simulink model "Unreal_Engine4"  (R2021a)
settings: Solver=ode14x  StartTime=0.0  StopTime=10.0  FixedStep=0.001  RelTol=1e-3
values from neighbouring files (symbols this model uses):
  env = read_environment_data    [main.m]
libraries: sim3dlib x28, simulink_extras x19, sim3dcameralib x1
settings Model: Creator=mojta  LastModifiedBy=mojta

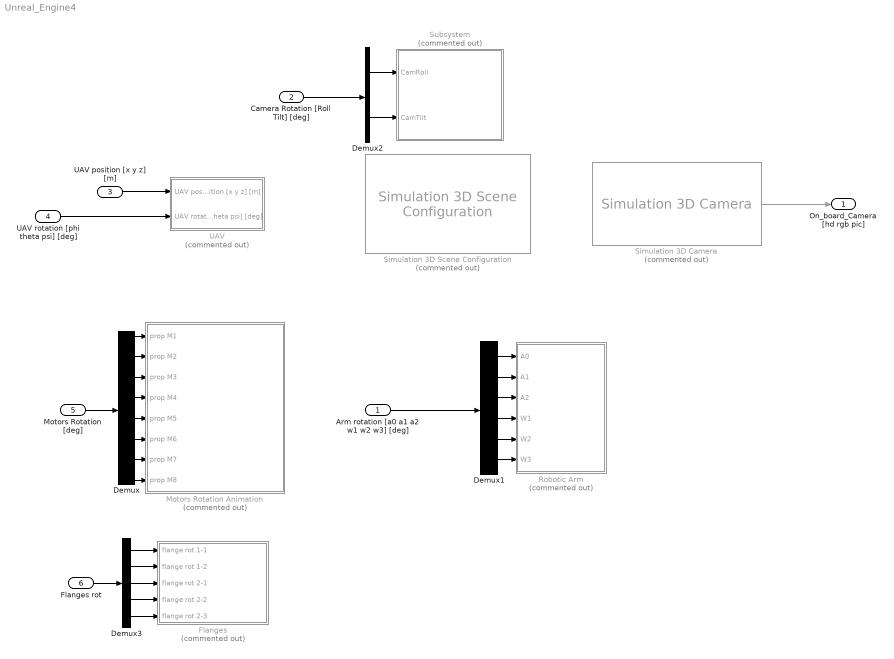
== system Unreal_Engine4 ==
  Arm rotation [a0 a1 a2 w1 w2 w3] [deg] : Inport  PortDimensions=6
  Camera Rotation [Roll Tilt] [deg] : Inport  Port=2  PortDimensions=2
  UAV position [x y z] [m] : Inport  Port=3  PortDimensions=3
  UAV rotation [phi theta psi] [deg] : Inport  Port=4  PortDimensions=3
  Motors Rotation [deg] : Inport  Port=5  PortDimensions=8
  Flanges rot : Inport  Port=6
  Demux : Demux  Outputs=8
  Demux1 : Demux  Outputs=6
  Demux2 : Demux  Outputs=2
  Demux3 : Demux  Outputs=5
  Flanges : Subsystem  Commented=on
  Motors Rotation Animation : Subsystem  Commented=on
  Robotic Arm : Subsystem  Commented=on
  Simulation 3D Camera : sim3dcameralib/Simulation 3D Camera  Priority=1  Commented=on  sensorTag=Sim3dSensor2  sensorId=2  sensorName=Sim3dSensor2  vehTagList={'Scene Origin'}  vehTag=Scene Origin  mountLoc=Origin  offsetFlag=on  tmountOffset=[0, 0, 0]  rmountOffset=[0 0 90]  FocalLength=[1109, 1109]  OpticalCenter=[640, 360]  ImageSize=[720, 1280]  RadialDistortion=[0, 0]  TangentialDistortion=[0, 0]  SensorSkew=0  DepthOutportEnabled=off  SemanticOutportEnabled=off  TransformOutportEnabled=off  SampleTime=1/160  mountPoint=[0 0 0]  mountOrientation=[0 0 -90]  aMode=3  ID=2
      settings: SourceProductBaseCode=DR,UV,VE
  Simulation 3D Scene Configuration : sim3dlib/Simulation 3D Scene Configuration  Priority=0  Commented=on  ProjectFormat=Unreal Editor  SceneDesc=Straight road  ProjectName=C:\Program Files\Polyspace\R2021a\toolbox\shared\sim3d_projects\automotive_project\UE4\WindowsNoEditor\VehicleSimulation.exe  ScenePath=/Game/Maps/HwStrght  UEProjPath=D:\MS_Control_Project\Sim_Env\Environment_1\Environment_1.uproject  vehTagList={'Scene Origin'}  vehTag=Scene Origin  OpVisEn=off  Ts=0.02  EnableWindow=on  EnableWeather=off  SunAltitude=40.0  SunAzimuth=90  clouds=10  wind=1  fog=0  rain=0  sensorTag=MainCamera1  sensorId=1  sensorName=MainCamera1  mountLoc=Origin  offsetFlag=off  tmountOffset=[0, 0, 0]  rmountOffset=[0, 0, 0]  HorizontalResolution=1280  VerticalResolution=720  HorizontalFOV=60  mountPoint=[0 0 0]  mountOrientation=[0 0 0]  aMode=2  ID=1
      settings: SourceProductBaseCode=DR,UV,VE
  Subsystem : Subsystem  Commented=on
  UAV : Subsystem  Commented=on
  On_board_Camera [hd rgb pic] : Outport  PortDimensions=[1280 720 3]
  wires:
  Simulation 3D Camera/1 -> On_board_Camera [hd rgb pic]/1
  Demux1/1 -> Robotic Arm/1(A0)
  Demux2/2 -> Subsystem/2(CamTilt)
  Demux1/3 -> Robotic Arm/3(A2)
  Demux1/5 -> Robotic Arm/5(W2)
  Demux2/1 -> Subsystem/1(CamRoll)
  Demux/5 -> Motors Rotation Animation/5(prop M5)
  Demux/7 -> Motors Rotation Animation/7(prop M7)
  Demux/3 -> Motors Rotation Animation/3(prop M3)
  Demux/1 -> Motors Rotation Animation/1(prop M1)
  Demux/2 -> Motors Rotation Animation/2(prop M2)
  Demux/4 -> Motors Rotation Animation/4(prop M4)
  Demux/6 -> Motors Rotation Animation/6(prop M6)
  Demux/8 -> Motors Rotation Animation/8(prop M8)
  Motors Rotation [deg]/1 -> Demux/1
  UAV position [x y z] [m]/1 -> UAV/1(UAV position [x y z] [m])
  UAV rotation [phi theta psi] [deg]/1 -> UAV/2(UAV rotation [phi theta psi] [deg])
  Demux1/2 -> Robotic Arm/2(A1)
  Demux1/4 -> Robotic Arm/4(W1)
  Demux1/6 -> Robotic Arm/6(W3)
  Arm rotation [a0 a1 a2 w1 w2 w3] [deg]/1 -> Demux1/1
  Camera Rotation [Roll Tilt] [deg]/1 -> Demux2/1
  Demux3/1 -> Flanges/1(flange rot 1-1)
  Demux3/2 -> Flanges/2(flange rot 1-2)
  Demux3/3 -> Flanges/3(flange rot 2-1)
  Demux3/4 -> Flanges/4(flange rot 2-2)
  Demux3/5 -> Flanges/5(flange rot 2-3)
  Flanges rot/1 -> Demux3/1

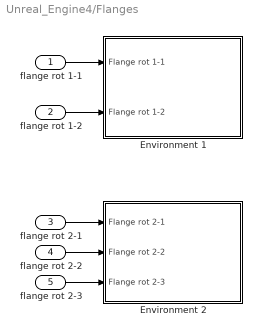
== system Unreal_Engine4/Flanges ==
  flange rot 1-1 : Inport  PortDimensions=8
  flange rot 1-2 : Inport  Port=2  PortDimensions=8
  flange rot 2-1 : Inport  Port=3  PortDimensions=6
  flange rot 2-2 : Inport  Port=4  PortDimensions=6
  flange rot 2-3 : Inport  Port=5  PortDimensions=6
  Environment 1 : Subsystem  TreatAsAtomicUnit=on
  Environment 2 : Subsystem  TreatAsAtomicUnit=on
  wires:
  flange rot 2-2/1 -> Environment 2/2(Flange rot 2-2)
  flange rot 2-3/1 -> Environment 2/3(Flange rot 2-3)
  flange rot 1-1/1 -> Environment 1/1(Flange rot 1-1)
  flange rot 1-2/1 -> Environment 1/2(Flange rot 1-2)
  flange rot 2-1/1 -> Environment 2/1(Flange rot 2-1)

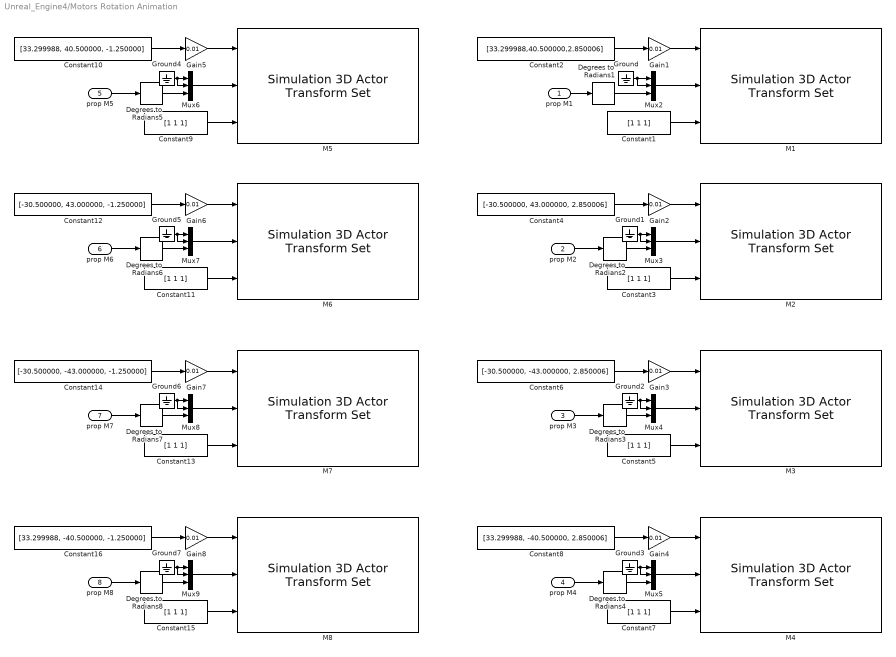
== system Unreal_Engine4/Motors Rotation Animation ==
  prop M1 : Inport
  prop M2 : Inport  Port=2
  prop M3 : Inport  Port=3
  prop M4 : Inport  Port=4
  prop M5 : Inport  Port=5
  prop M6 : Inport  Port=6
  prop M7 : Inport  Port=7
  prop M8 : Inport  Port=8
  Constant{1,3,5,7,9,11,13,15} (8 alike) : Constant  Value=[1 1 1]
  Constant10 : Constant  Value=[33.299988, 40.500000, -1.250000]
  Constant12 : Constant  Value=[-30.500000, 43.000000, -1.250000]
  Constant14 : Constant  Value=[-30.500000, -43.000000, -1.250000]
  Constant16 : Constant  Value=[33.299988, -40.500000, -1.250000]
  Constant2 : Constant  Value=[33.299988,40.500000,2.850006]
  Constant4 : Constant  Value=[-30.500000, 43.000000, 2.850006]
  Constant6 : Constant  Value=[-30.500000, -43.000000, 2.850006]
  Constant8 : Constant  Value=[33.299988, -40.500000, 2.850006]
  Degrees to Radians{1..8} (8 alike) : simulink_extras/Transformations/Degrees to Radians
  Gain{1..8} (8 alike) : Gain  Gain=0.01
  Ground{,1..7} (8 alike) : Ground
  M1 : sim3dlib/Simulation 3D Actor Transform Set  Priority=-1  ActorTag=M1  NumberOfParts=1  CustNumOfParts=3  Translation=[0 0 0]  Rotation=[0 0 0]  Scale=[1 1 1]  Ts=-1  aMode=2
      settings: SourceProductBaseCode=DR,UV,VE
  M2 : sim3dlib/Simulation 3D Actor Transform Set  Priority=-1  ActorTag=M2  NumberOfParts=1  CustNumOfParts=3  Translation=[0 0 0]  Rotation=[0 0 0]  Scale=[1 1 1]  Ts=-1  aMode=2
      settings: SourceProductBaseCode=DR,UV,VE
  M3 : sim3dlib/Simulation 3D Actor Transform Set  Priority=-1  ActorTag=M3  NumberOfParts=1  CustNumOfParts=3  Translation=[0 0 0]  Rotation=[0 0 0]  Scale=[1 1 1]  Ts=-1  aMode=2
      settings: SourceProductBaseCode=DR,UV,VE
  M4 : sim3dlib/Simulation 3D Actor Transform Set  Priority=-1  ActorTag=M4  NumberOfParts=1  CustNumOfParts=3  Translation=[0 0 0]  Rotation=[0 0 0]  Scale=[1 1 1]  Ts=-1  aMode=2
      settings: SourceProductBaseCode=DR,UV,VE
  M5 : sim3dlib/Simulation 3D Actor Transform Set  Priority=-1  ActorTag=M5  NumberOfParts=1  CustNumOfParts=3  Translation=[0 0 0]  Rotation=[0 0 0]  Scale=[1 1 1]  Ts=-1  aMode=2
      settings: SourceProductBaseCode=DR,UV,VE
  M6 : sim3dlib/Simulation 3D Actor Transform Set  Priority=-1  ActorTag=M6  NumberOfParts=1  CustNumOfParts=3  Translation=[0 0 0]  Rotation=[0 0 0]  Scale=[1 1 1]  Ts=-1  aMode=2
      settings: SourceProductBaseCode=DR,UV,VE
  M7 : sim3dlib/Simulation 3D Actor Transform Set  Priority=-1  ActorTag=M7  NumberOfParts=1  CustNumOfParts=3  Translation=[0 0 0]  Rotation=[0 0 0]  Scale=[1 1 1]  Ts=-1  aMode=2
      settings: SourceProductBaseCode=DR,UV,VE
  M8 : sim3dlib/Simulation 3D Actor Transform Set  Priority=-1  ActorTag=M8  NumberOfParts=1  CustNumOfParts=3  Translation=[0 0 0]  Rotation=[0 0 0]  Scale=[1 1 1]  Ts=-1  aMode=2
      settings: SourceProductBaseCode=DR,UV,VE
  Mux{2..9} (8 alike) : Mux  Inputs=3
  wires:
  Ground7/1 -> Mux9/1, Mux9/2
  Mux9/1 -> M8/2
  Constant7/1 -> M4/3
  Constant1/1 -> M1/3
  Gain8/1 -> M8/1
  Constant15/1 -> M8/3
  Constant16/1 -> Gain8/1
  Ground5/1 -> Mux7/2, Mux7/1
  prop M5/1 -> Degrees to Radians5/1
  Constant12/1 -> Gain6/1
  Constant6/1 -> Gain3/1
  prop M7/1 -> Degrees to Radians7/1
  Degrees to Radians1/1 -> Mux2/3
  Mux5/1 -> M4/2
  prop M2/1 -> Degrees to Radians2/1
  prop M4/1 -> Degrees to Radians4/1
  Gain7/1 -> M7/1
  Constant11/1 -> M6/3
  Degrees to Radians7/1 -> Mux8/3
  Mux8/1 -> M7/2
  Degrees to Radians6/1 -> Mux7/3
  Constant5/1 -> M3/3
  Mux4/1 -> M3/2
  Constant13/1 -> M7/3
  Gain1/1 -> M1/1
  Mux7/1 -> M6/2
  prop M3/1 -> Degrees to Radians3/1
  Constant14/1 -> Gain7/1
  prop M6/1 -> Degrees to Radians6/1
  Mux6/1 -> M5/2
  Gain6/1 -> M6/1
  Gain5/1 -> M5/1
  Degrees to Radians5/1 -> Mux6/3
  Degrees to Radians2/1 -> Mux3/3
  Gain3/1 -> M3/1
  Constant10/1 -> Gain5/1
  Constant8/1 -> Gain4/1
  Constant9/1 -> M5/3
  Constant4/1 -> Gain2/1
  Ground1/1 -> Mux3/2, Mux3/1
  Ground6/1 -> Mux8/1, Mux8/2
  Constant2/1 -> Gain1/1
  Ground4/1 -> Mux6/2, Mux6/1
  Ground3/1 -> Mux5/2, Mux5/1
  Ground/1 -> Mux2/2, Mux2/1
  Constant3/1 -> M2/3
  Ground2/1 -> Mux4/2, Mux4/1
  prop M8/1 -> Degrees to Radians8/1
  Mux3/1 -> M2/2
  Gain2/1 -> M2/1
  prop M1/1 -> Degrees to Radians1/1
  Mux2/1 -> M1/2
  Gain4/1 -> M4/1
  Degrees to Radians8/1 -> Mux9/3
  Degrees to Radians3/1 -> Mux4/3
  Degrees to Radians4/1 -> Mux5/3

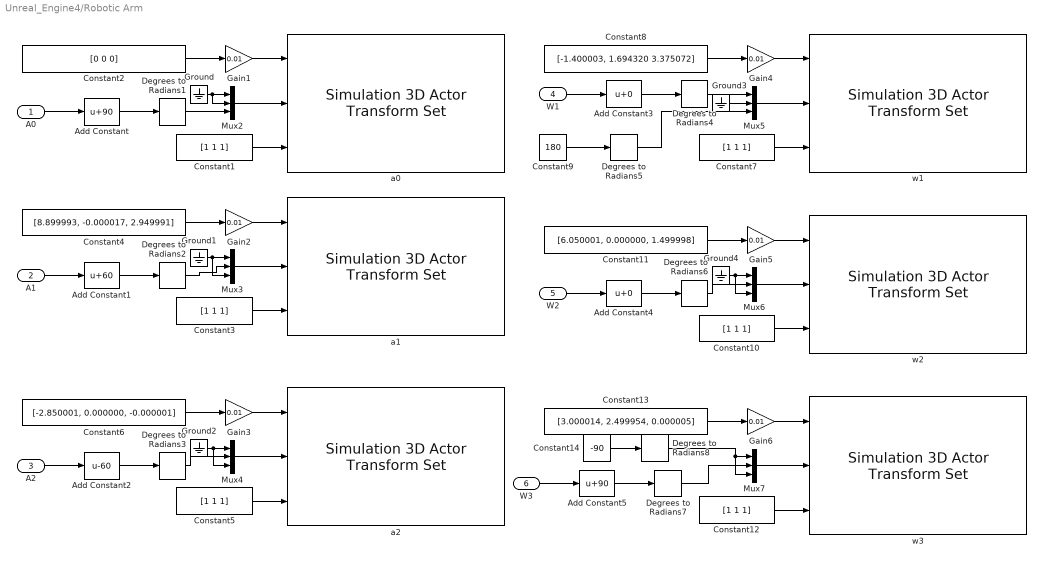
== system Unreal_Engine4/Robotic Arm ==
  A0 : Inport
  A1 : Inport  Port=2
  A2 : Inport  Port=3
  W1 : Inport  Port=4
  W2 : Inport  Port=5
  W3 : Inport  Port=6
  Add Constant : Bias  Bias=90
  Add Constant1 : Bias  Bias=60
  Add Constant2 : Bias  Bias=-60
  Add Constant3 : Bias
  Add Constant4 : Bias
  Add Constant5 : Bias  Bias=90
  Constant{1,3,5,7,10,12} (6 alike) : Constant  Value=[1 1 1]
  Constant11 : Constant  Value=[6.050001, 0.000000, 1.499998]
  Constant13 : Constant  Value=[3.000014, 2.499954, 0.000005]
  Constant14 : Constant  Value=-90
  Constant2 : Constant  Value=[0 0 0]
  Constant4 : Constant  Value=[8.899993, -0.000017, 2.949991]
  Constant6 : Constant  Value=[-2.850001, 0.000000, -0.000001]
  Constant8 : Constant  Value=[-1.400003, 1.694320 3.375072]
  Constant9 : Constant  Value=180
  Degrees to Radians{1..8} (8 alike) : simulink_extras/Transformations/Degrees to Radians
  Gain{1..6} (6 alike) : Gain  Gain=0.01
  Ground{,1..4} (5 alike) : Ground
  Mux{2..7} (6 alike) : Mux  Inputs=3
  a0 : sim3dlib/Simulation 3D Actor Transform Set  Priority=-1  ActorTag=A0  NumberOfParts=1  CustNumOfParts=3  Translation=[0 0 0]  Rotation=[0 0 0]  Scale=[1 1 1]  Ts=-1  aMode=2
      settings: SourceProductBaseCode=DR,UV,VE
  a1 : sim3dlib/Simulation 3D Actor Transform Set  Priority=-1  ActorTag=A1  NumberOfParts=1  CustNumOfParts=3  Translation=[0 0 0]  Rotation=[0 0 0]  Scale=[1 1 1]  Ts=-1  aMode=2
      settings: SourceProductBaseCode=DR,UV,VE
  a2 : sim3dlib/Simulation 3D Actor Transform Set  Priority=-1  ActorTag=A2  NumberOfParts=1  CustNumOfParts=3  Translation=[0 0 0]  Rotation=[0 0 0]  Scale=[1 1 1]  Ts=-1  aMode=2
      settings: SourceProductBaseCode=DR,UV,VE
  w1 : sim3dlib/Simulation 3D Actor Transform Set  Priority=-1  ActorTag=W1  NumberOfParts=1  CustNumOfParts=3  Translation=[0 0 0]  Rotation=[0 0 0]  Scale=[1 1 1]  Ts=-1  aMode=2
      settings: SourceProductBaseCode=DR,UV,VE
  w2 : sim3dlib/Simulation 3D Actor Transform Set  Priority=-1  ActorTag=W2  NumberOfParts=1  CustNumOfParts=3  Translation=[0 0 0]  Rotation=[0 0 0]  Scale=[1 1 1]  Ts=-1  aMode=2
      settings: SourceProductBaseCode=DR,UV,VE
  w3 : sim3dlib/Simulation 3D Actor Transform Set  Priority=-1  ActorTag=W3  NumberOfParts=1  CustNumOfParts=3  Translation=[0 0 0]  Rotation=[0 0 0]  Scale=[1 1 1]  Ts=-1  aMode=2
      settings: SourceProductBaseCode=DR,UV,VE
  wires:
  Constant7/1 -> w1/3
  Degrees to Radians2/1 -> Mux3/2
  W1/1 -> Add Constant3/1
  Mux3/1 -> a1/2
  Ground3/1 -> Mux5/2
  Constant14/1 -> Degrees to Radians8/1
  Gain4/1 -> w1/1
  Constant9/1 -> Degrees to Radians5/1
  Ground/1 -> Mux2/2, Mux2/1
  Degrees to Radians4/1 -> Mux5/1
  Constant8/1 -> Gain4/1
  Add Constant3/1 -> Degrees to Radians4/1
  Mux5/1 -> w1/2
  Mux7/1 -> w3/2
  Constant2/1 -> Gain1/1
  Degrees to Radians8/1 -> Mux7/1, Mux7/3
  Degrees to Radians1/1 -> Mux2/3
  Add Constant/1 -> Degrees to Radians1/1
  Constant1/1 -> a0/3
  Constant5/1 -> a2/3
  Mux6/1 -> w2/2
  Constant6/1 -> Gain3/1
  Mux2/1 -> a0/2
  Gain1/1 -> a0/1
  W2/1 -> Add Constant4/1
  Ground4/1 -> Mux6/3, Mux6/1
  Constant4/1 -> Gain2/1
  Constant11/1 -> Gain5/1
  Constant3/1 -> a1/3
  Add Constant4/1 -> Degrees to Radians6/1
  Mux4/1 -> a2/2
  Constant12/1 -> w3/3
  Degrees to Radians7/1 -> Mux7/2
  Constant13/1 -> Gain6/1
  W3/1 -> Add Constant5/1
  Add Constant2/1 -> Degrees to Radians3/1
  Gain6/1 -> w3/1
  Add Constant5/1 -> Degrees to Radians7/1
  A0/1 -> Add Constant/1
  Degrees to Radians3/1 -> Mux4/2
  A2/1 -> Add Constant2/1
  Gain5/1 -> w2/1
  Add Constant1/1 -> Degrees to Radians2/1
  Constant10/1 -> w2/3
  Gain2/1 -> a1/1
  Ground1/1 -> Mux3/3, Mux3/1
  Degrees to Radians5/1 -> Mux5/3
  Ground2/1 -> Mux4/3, Mux4/1
  Gain3/1 -> a2/1
  A1/1 -> Add Constant1/1
  Degrees to Radians6/1 -> Mux6/2

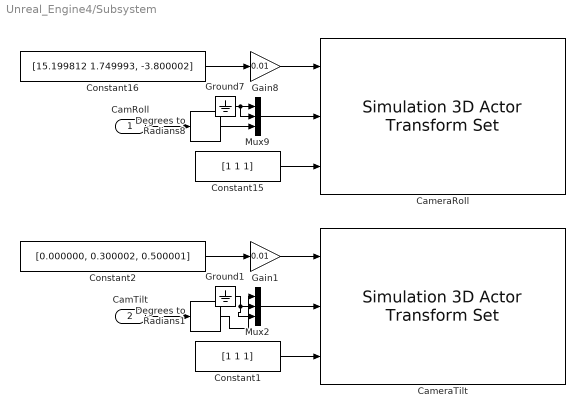
== system Unreal_Engine4/Subsystem ==
  CamRoll : Inport
  CamTilt : Inport  Port=2
  CameraRoll : sim3dlib/Simulation 3D Actor Transform Set  Priority=-1  ActorTag=CamRoll  NumberOfParts=1  CustNumOfParts=3  Translation=[0 0 0]  Rotation=[0 0 0]  Scale=[1 1 1]  Ts=-1  aMode=2
      settings: SourceProductBaseCode=DR,UV,VE
  CameraTilt : sim3dlib/Simulation 3D Actor Transform Set  Priority=-1  ActorTag=CamTilt  NumberOfParts=1  CustNumOfParts=3  Translation=[0 0 0]  Rotation=[0 0 0]  Scale=[1 1 1]  Ts=-1  aMode=2
      settings: SourceProductBaseCode=DR,UV,VE
  Constant1 : Constant  Value=[1 1 1]
  Constant15 : Constant  Value=[1 1 1]
  Constant16 : Constant  Value=[15.199812 1.749993, -3.800002]
  Constant2 : Constant  Value=[0.000000, 0.300002, 0.500001]
  Degrees to Radians1 : simulink_extras/Transformations/Degrees to Radians
  Degrees to Radians8 : simulink_extras/Transformations/Degrees to Radians
  Gain1 : Gain  Gain=0.01
  Gain8 : Gain  Gain=0.01
  Ground1 : Ground
  Ground7 : Ground
  Mux2 : Mux  Inputs=3
  Mux9 : Mux  Inputs=3
  wires:
  Gain1/1 -> CameraTilt/1
  Constant15/1 -> CameraRoll/3
  Constant16/1 -> Gain8/1
  Ground1/1 -> Mux2/2, Mux2/3
  Gain8/1 -> CameraRoll/1
  Constant1/1 -> CameraTilt/3
  Ground7/1 -> Mux9/1, Mux9/2
  Degrees to Radians8/1 -> Mux9/3
  Mux9/1 -> CameraRoll/2
  CamRoll/1 -> Degrees to Radians8/1
  CamTilt/1 -> Degrees to Radians1/1
  Constant2/1 -> Gain1/1
  Mux2/1 -> CameraTilt/2
  Degrees to Radians1/1 -> Mux2/1

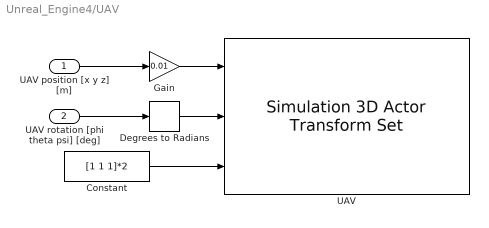
== system Unreal_Engine4/UAV ==
  UAV position [x y z] [m] : Inport
  UAV rotation [phi theta psi] [deg] : Inport  Port=2
  Constant : Constant  Value=[1 1 1]*2
  Degrees to Radians : simulink_extras/Transformations/Degrees to Radians
  Gain : Gain  Gain=0.01
  UAV : sim3dlib/Simulation 3D Actor Transform Set  Priority=-1  ActorTag=uav  NumberOfParts=1  CustNumOfParts=3  Translation=[0 0 0]  Rotation=[0 0 0]  Scale=[1 1 1]  Ts=-1  aMode=2
      settings: SourceProductBaseCode=DR,UV,VE
  wires:
  UAV position [x y z] [m]/1 -> Gain/1
  UAV rotation [phi theta psi] [deg]/1 -> Degrees to Radians/1
  Degrees to Radians/1 -> UAV/2
  Gain/1 -> UAV/1
  Constant/1 -> UAV/3

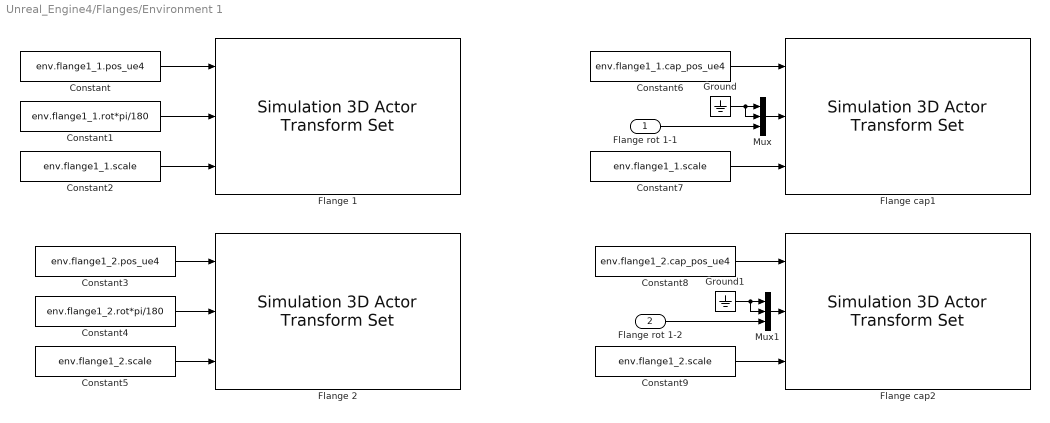
== system Unreal_Engine4/Flanges/Environment 1 ==
  Flange rot 1-1 : Inport
  Flange rot 1-2 : Inport  Port=2
  Constant : Constant  Value=env.flange1_1.pos_ue4
  Constant1 : Constant  Value=env.flange1_1.rot*pi/180
  Constant2 : Constant  Value=env.flange1_1.scale
  Constant3 : Constant  Value=env.flange1_2.pos_ue4
  Constant4 : Constant  Value=env.flange1_2.rot*pi/180
  Constant5 : Constant  Value=env.flange1_2.scale
  Constant6 : Constant  Value=env.flange1_1.cap_pos_ue4
  Constant7 : Constant  Value=env.flange1_1.scale
  Constant8 : Constant  Value=env.flange1_2.cap_pos_ue4
  Constant9 : Constant  Value=env.flange1_2.scale
  Flange 1 : sim3dlib/Simulation 3D Actor Transform Set  Priority=-1  ActorTag=flange1_1  NumberOfParts=1  CustNumOfParts=3  Translation=[0 0 0]  Rotation=[0 0 0]  Scale=[1 1 1]  Ts=-1  aMode=2
      settings: SourceProductBaseCode=DR,UV,VE
  Flange 2 : sim3dlib/Simulation 3D Actor Transform Set  Priority=-1  ActorTag=flange1_2  NumberOfParts=1  CustNumOfParts=3  Translation=[0 0 0]  Rotation=[0 0 0]  Scale=[1 1 1]  Ts=-1  aMode=2
      settings: SourceProductBaseCode=DR,UV,VE
  Flange cap1 : sim3dlib/Simulation 3D Actor Transform Set  Priority=-1  ActorTag=flange_cap1_1  NumberOfParts=1  CustNumOfParts=3  Translation=[0 0 0]  Rotation=[0 0 0]  Scale=[1 1 1]  Ts=-1  aMode=2
      settings: SourceProductBaseCode=DR,UV,VE
  Flange cap2 : sim3dlib/Simulation 3D Actor Transform Set  Priority=-1  ActorTag=flangecap1_2  NumberOfParts=1  CustNumOfParts=3  Translation=[0 0 0]  Rotation=[0 0 0]  Scale=[1 1 1]  Ts=-1  aMode=2
      settings: SourceProductBaseCode=DR,UV,VE
  Ground : Ground
  Ground1 : Ground
  Mux : Mux  Inputs=3
  Mux1 : Mux  Inputs=3
  wires:
  Constant/1 -> Flange 1/1
  Constant1/1 -> Flange 1/2
  Constant2/1 -> Flange 1/3
  Constant3/1 -> Flange 2/1
  Constant4/1 -> Flange 2/2
  Constant5/1 -> Flange 2/3
  Constant6/1 -> Flange cap1/1
  Constant7/1 -> Flange cap1/3
  Mux/1 -> Flange cap1/2
  Flange rot 1-1/1 -> Mux/3
  Ground/1 -> Mux/2, Mux/1
  Ground1/1 -> Mux1/1, Mux1/2
  Flange rot 1-2/1 -> Mux1/3
  Mux1/1 -> Flange cap2/2
  Constant9/1 -> Flange cap2/3
  Constant8/1 -> Flange cap2/1

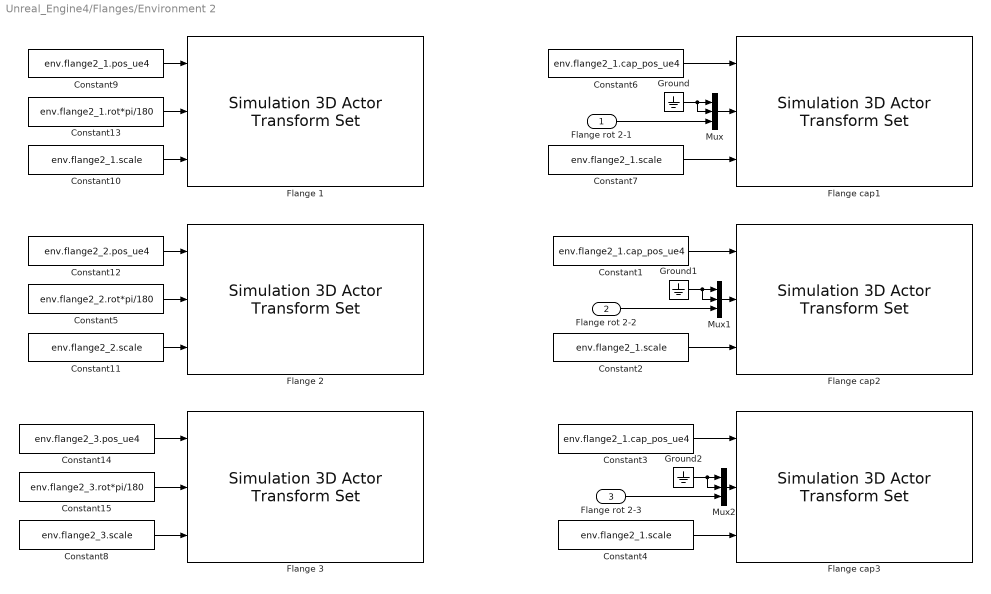
== system Unreal_Engine4/Flanges/Environment 2 ==
  Flange rot 2-1 : Inport
  Flange rot 2-2 : Inport  Port=2
  Flange rot 2-3 : Inport  Port=3
  Constant1 : Constant  Value=env.flange2_1.cap_pos_ue4
  Constant{2,4,7,10} (4 alike) : Constant  Value=env.flange2_1.scale
  Constant11 : Constant  Value=env.flange2_2.scale
  Constant12 : Constant  Value=env.flange2_2.pos_ue4
  Constant13 : Constant  Value=env.flange2_1.rot*pi/180
  Constant14 : Constant  Value=env.flange2_3.pos_ue4
  Constant15 : Constant  Value=env.flange2_3.rot*pi/180
  Constant3 : Constant  Value=env.flange2_1.cap_pos_ue4
  Constant5 : Constant  Value=env.flange2_2.rot*pi/180
  Constant6 : Constant  Value=env.flange2_1.cap_pos_ue4
  Constant8 : Constant  Value=env.flange2_3.scale
  Constant9 : Constant  Value=env.flange2_1.pos_ue4
  Flange 1 : sim3dlib/Simulation 3D Actor Transform Set  Priority=-1  ActorTag=flange2_1  NumberOfParts=1  CustNumOfParts=3  Translation=[0 0 0]  Rotation=[0 0 0]  Scale=[1 1 1]  Ts=-1  aMode=2
      settings: SourceProductBaseCode=DR,UV,VE
  Flange 2 : sim3dlib/Simulation 3D Actor Transform Set  Priority=-1  ActorTag=flange2_2  NumberOfParts=1  CustNumOfParts=3  Translation=[0 0 0]  Rotation=[0 0 0]  Scale=[1 1 1]  Ts=-1  aMode=2
      settings: SourceProductBaseCode=DR,UV,VE
  Flange 3 : sim3dlib/Simulation 3D Actor Transform Set  Priority=-1  ActorTag=flnage2_3  NumberOfParts=1  CustNumOfParts=3  Translation=[0 0 0]  Rotation=[0 0 0]  Scale=[1 1 1]  Ts=-1  aMode=2
      settings: SourceProductBaseCode=DR,UV,VE
  Flange cap1 : sim3dlib/Simulation 3D Actor Transform Set  Priority=-1  ActorTag=flangecap2_1  NumberOfParts=1  CustNumOfParts=3  Translation=[0 0 0]  Rotation=[0 0 0]  Scale=[1 1 1]  Ts=-1  aMode=2
      settings: SourceProductBaseCode=DR,UV,VE
  Flange cap2 : sim3dlib/Simulation 3D Actor Transform Set  Priority=-1  ActorTag=flangecap2_2  NumberOfParts=1  CustNumOfParts=3  Translation=[0 0 0]  Rotation=[0 0 0]  Scale=[1 1 1]  Ts=-1  aMode=2
      settings: SourceProductBaseCode=DR,UV,VE
  Flange cap3 : sim3dlib/Simulation 3D Actor Transform Set  Priority=-1  ActorTag=flangecap2_3  NumberOfParts=1  CustNumOfParts=3  Translation=[0 0 0]  Rotation=[0 0 0]  Scale=[1 1 1]  Ts=-1  aMode=2
      settings: SourceProductBaseCode=DR,UV,VE
  Ground : Ground
  Ground1 : Ground
  Ground2 : Ground
  Mux : Mux  Inputs=3
  Mux1 : Mux  Inputs=3
  Mux2 : Mux  Inputs=3
  wires:
  Flange rot 2-1/1 -> Mux/3
  Constant7/1 -> Flange cap1/3
  Ground/1 -> Mux/2, Mux/1
  Constant6/1 -> Flange cap1/1
  Mux/1 -> Flange cap1/2
  Mux1/1 -> Flange cap2/2
  Constant1/1 -> Flange cap2/1
  Ground1/1 -> Mux1/1, Mux1/2
  Constant2/1 -> Flange cap2/3
  Flange rot 2-2/1 -> Mux1/3
  Flange rot 2-3/1 -> Mux2/3
  Constant4/1 -> Flange cap3/3
  Ground2/1 -> Mux2/2, Mux2/1
  Constant3/1 -> Flange cap3/1
  Mux2/1 -> Flange cap3/2
  Constant14/1 -> Flange 3/1
  Constant8/1 -> Flange 3/3
  Constant10/1 -> Flange 1/3
  Constant9/1 -> Flange 1/1
  Constant12/1 -> Flange 2/1
  Constant11/1 -> Flange 2/3
  Constant13/1 -> Flange 1/2
  Constant5/1 -> Flange 2/2
  Constant15/1 -> Flange 3/2
